simulink model "Robo_Bipede_Contato"  (R2020a)
settings: Solver=ode15s  StartTime=0.0  StopTime=1  MaxStep=1e-4  RelTol=1e-4  AbsTol=1e-5  EnableMultiTasking=on
model workspace: external: MATLAB File C:\Users\LUIS IZQUIERDO C\Desktop\PROGRAMAS TESE\13. ROBO BIPEDE SIMSCAPE COM CONTATO\Model_Params_Contato.m (data not in the file)
values from neighbouring files (symbols this model uses):
  CoG_y = 0.091733    [Model_Params_Cont_FSM.m]
  height_plane = 0.025    [Model_Params_Cont_FSM.m]
  m_esfera = 1    [Model_Params_Cont_FSM.m]
  plane_height = height_plane    (= 0.025)    [Model_Params_Cont_FSM.m]
  plane_length = 50    [Model_Params_Cont_FSM.m]
  plane_width = 3    [Model_Params_Cont_FSM.m]
  temp = Dados_XY1_D(ciclo,1)    [Model_Params_Cont_FSM.m]
  velocidade = 1    [Model_Params_Cont_FSM.m]
  Xpq2_D = Xpq2_D'    [Model_Params_Cont_FSM.m]
  Xpq3_D = Xpq3_D'    [Model_Params_Cont_FSM.m]
  Ypq2_D = Ypq2_D'    [Model_Params_Cont_FSM.m]
  Ypq3_D = Ypq3_D'    [Model_Params_Cont_FSM.m]
undefined symbols (not defined in the file or in its folder): COXA, HAT, PE, PERNA, X, Y, Z
libraries: nesl_utility x70, sm_lib x61, simulink x1
(part 3 of 3)

== stateflow chart Robo_Bipede_Contato/Chart ==
  settings: updateMethod=DISCRETE  sampleTime=0.002
  state FSM4EV/
    entry:
    theta0_right=[deg2rad(25.6131); deg2rad(14.72863); deg2rad(0.0003)];
    theta0_left=[deg2rad(-9.8611); deg2rad(25.8751); deg2rad(12.74498)];
    Count=1;
    HS1E=0;
    TO1D=0;
    HS2D=0;
    TO2E=0;
    during:
    if Count ~= 100
    Count = Count +1
    else
    Count = 1;
    end
    state ADBE/
      during:
      XqpD = Trajectory1(1,Count) - Trajectory1(3,Count);
      YqpD = Trajectory1(2,Count) - Trajectory1(4,Count);
      XpqE = Trajectory1(7,Count) - Trajectory1(5,Count);
      YpqE = Trajectory1(8,Count) - Trajectory1(6,Count);
      Traj_STR = [ XqpD; YqpD;0];
      Traj_SW = [XpqE; YpqE;0];
      theta_right=Inv_Kinem_Stance(Traj_STR, theta0_right);
      theta_left=Inv_Kinem_Swing(Traj_SW, theta0_left);
      theta0_right=theta_right;
      theta0_left=theta_left;
      if Count==45
      HS1E=1;
      TO2E=0;
      end
    state ADE/
      during:
      XqpD = Trajectory1(1,Count) - Trajectory1(3,Count);
      YqpD = Trajectory1(2,Count)  - Trajectory1(4,Count);
      XqpE = Trajectory1(5,Count) - Trajectory1(7,Count);
      YqpE = Trajectory1(6,Count) - Trajectory1(8,Count);
      Traj_STR=[ XqpD; YqpD;0];
      Traj_STL=[XqpE;  YqpE;0];
      theta_right=Inv_Kinem_Stance(Traj_STR,theta0_right);
      theta_left=Inv_Kinem_Stance(Traj_STL,theta0_left);
      theta0_right=theta_right;
      theta0_left=theta_left;
      if Count==54
      TO1D=1;
      HS1E=0;
      end
    state BDAE/
      during:
      XpqD = Trajectory1(3,Count) - Trajectory1(1,Count);
      YpqD = Trajectory1(4,Count) - Trajectory1(2,Count);
      XqpE = Trajectory1(5,Count) - Trajectory1(7,Count);
      YqpE = Trajectory1(6,Count) - Trajectory1(8,Count);
      Traj_SW = [XpqD;  YpqD;0];
      Traj_STL=[ XqpE; YqpE;0];
      theta_right=Inv_Kinem_Swing(Traj_SW,theta0_right);
      theta_left=Inv_Kinem_Stance(Traj_STL,theta0_left);
      theta0_right=theta_right;
      theta0_left=theta_left;
      if Count==97
      HS2D=1;
      TO1D=0;
      end
    state ADD/
      during:
      XqpD = Trajectory1(1,Count) - Trajectory1(3,Count);
      YqpD = Trajectory1(2,Count)  - Trajectory1(4,Count);
      XqpE = Trajectory1(5,Count) - Trajectory1(7,Count);
      YqpE = Trajectory1(6,Count) - Trajectory1(8,Count);
      Traj_STR=[ XqpD; YqpD;0];
      Traj_STL=[XqpE;  YqpE;0];
      theta_right=Inv_Kinem_Stance(Traj_STR,theta0_right);
      theta_left=Inv_Kinem_Stance(Traj_STL,theta0_left);
      theta0_right=theta_right;
      theta0_left=theta_left;
      if Count==100
      TO2E=1;
      HS2D=0;
      end
    (default) -> ADBE
    ADBE -> ADE : [HS1E==1]
    ADD -> ADBE : [TO2E==1]
    ADE -> BDAE : [TO1D==1]
    BDAE -> ADD : [HS2D==1]
  (default) -> FSM4EV
  data: Ptraj function_input; theta_ini function_input; theta_swing function_output; Ptraj function_input; theta_ini function_input; theta_stance function_output; tempo input; Trajectory1 input; Trajectory2 input; Trajectory3 input; Count local; V input; HS1E local double; TO1D local double; HS2D local double; TO2E local double; XqtD local double; YqtD local double; XtqD local double; YtqD local double; XtqE local double; YtqE local double; XqtE local double; YqtE local double; Traj_SW local size=[3,1]; Traj_STR local size=[3,1]; Traj_STL local size=[3,1]; theta_right output size=[3,1]; theta_left output size=[3,1]; theta0_right local size=[3,1]; theta0_left local size=[3,1]; XpqD local; XpqE local; XqpD local; XqpE local; YpqD local; YpqE local; YqpD local; YqpE local; FcDi input; Pospe_Di input; FcEi input; Pospe_Ei input; ChartMode output Enum: ChartModeType
  function theta_swing = Inv_Kinem_Swing(Ptraj,theta_ini):
    | function theta_swing = Inv_Kinem_Swing(Ptraj,theta_ini)
    | 
    | %% CINEMÁTICA INVERSA PARA A FASE DE BALANCO
    | 
    | Lc = 0.42;     % Comprimento coxa (m)
    | Lj = 0.46;     % Comprimento da perna (m)
    | % Lp = 0.153;  % Comprimento do pe(m) 
    | Lp = 0.10;     % Comprimento do pe(m)
    | H = 1.72;      % Altura da pessoa
    | a0 = 0;
    | d0 = 0.19*H/2; % metade da largura do HAT
    | 
    | % Vetor de angulos iniciais theta_ini = [theta_q; theta_j]
    | theta_q = theta_ini(1);
    | theta_j = theta_ini(2);
    | theta_t = theta_ini(3);
    | 
    | %% EQUACOES DA CINEMATICA DIRETA
    | %Posicao do dedao em relacao a junta do quadril (FASE BALANCO)
    | P_ini =[Lc*sin(theta_q) + Lj*sin(theta_q - theta_j) + Lp*cos(theta_q - theta_j + theta_t); 
    |        -Lc*cos(theta_q) - Lj*cos(theta_q - theta_j) + Lp*sin(theta_q - theta_j + theta_t); 
    |         0];
    | 
    | 
    | %% EQUACOES DA CINEMATICA INVERSA
    | %Matriz Jacobiana Inversa J^-1 Fase de Balanco
    | % determ = Lc*Lj*sj;
    | % Jinv = (1/determ)*[-Lj*sqj, Lj*cqj; -(Lc*sq+Lj*sqj), Lc*cq+Lj*cqj];
    | 
    | tht_1 = theta_q;
    | tht_2 = theta_j;
    | tht_3 = theta_t;
    | 
    | Jinv_bal3gl = zeros(3,3);
    | 
    | Jinv_bal3gl(1,1) = (Lc*Lj^2*cos(tht_1) + 2*Lc*Lp^2*cos(tht_1) +...
    |     2*Lc*Lp^2*cos(tht_1 - 2*tht_2 + 2*tht_3) + Lj*Lp^2*cos(tht_1 - tht_2 + 2*tht_3) -...
    |     Lc*Lj^2*cos(tht_1 - 2*tht_2) + Lj*Lp^2*cos(tht_1 - tht_2) -...
    |     Lc*Lj*Lp*sin(tht_1 + tht_3) + Lc*Lj*Lp*sin(tht_1 - tht_3) +...
    |     2*Lc*Lj*Lp*sin(tht_1 - 2*tht_2 + tht_3))/(Lc^2*Lj^2 + 2*Lc^2*Lp^2 + 2*Lj^2*Lp^2 +...
    |     2*Lc^2*Lp^2*cos(2*tht_2 - 2*tht_3) - Lc^2*Lj^2*cos(2*tht_2) + 2*Lj^2*Lp^2*cos(2*tht_3) -...
    |     2*Lc^2*Lj*Lp*sin(2*tht_2 - tht_3) + 2*Lc*Lj*Lp^2*cos(tht_2) - 2*Lc^2*Lj*Lp*sin(tht_3) +...
    |     2*Lc*Lj*Lp^2*cos(tht_2 - 2*tht_3));
    | 
    | Jinv_bal3gl(2,1) = (Lc^2*Lj*cos(tht_1 + tht_2) + Lc*Lj^2*cos(tht_1) + Lc*Lp^2*cos(tht_1) +...
    |     Lc*Lp^2*cos(tht_1 - 2*tht_2 + 2*tht_3) - Lj*Lp^2*cos(tht_1 - tht_2 + 2*tht_3) -...
    |     Lc^2*Lj*cos(tht_1 - tht_2) - Lc*Lj^2*cos(tht_1 - 2*tht_2) - Lj*Lp^2*cos(tht_1 - tht_2) +...
    |     Lc^2*Lp*sin(tht_1 + tht_2 - tht_3) + Lc^2*Lp*sin(tht_1 - tht_2 + tht_3) -...
    |     Lc*Lj*Lp*sin(tht_1 + tht_3) + Lc*Lj*Lp*sin(tht_1 - tht_3) +...
    |     2*Lc*Lj*Lp*sin(tht_1 - 2*tht_2 + tht_3))/(Lc^2*Lj^2 + 2*Lc^2*Lp^2 + 2*Lj^2*Lp^2 +...
    |     2*Lc^2*Lp^2*cos(2*tht_2 - 2*tht_3) - Lc^2*Lj^2*cos(2*tht_2) + 2*Lj^2*Lp^2*cos(2*tht_3) -...
    |     2*Lc^2*Lj*Lp*sin(2*tht_2 - tht_3) + 2*Lc*Lj*Lp^2*cos(tht_2) - 2*Lc^2*Lj*Lp*sin(tht_3) +...
    |     2*Lc*Lj*Lp^2*cos(tht_2 - 2*tht_3));
    | 
    | Jinv_bal3gl(3,1) = -(Lp*(Lc^2*sin(tht_1 + tht_2 - tht_3) + Lc^2*sin(tht_1 - tht_2 + tht_3) +...
    |     2*Lj^2*sin(tht_1 - tht_2 + tht_3) - 2*Lj^2*sin(tht_2 - tht_1 + tht_3) +...
    |     2*Lj*Lp*cos(tht_1 - tht_2) + 2*Lc*Lj*sin(tht_1 - tht_3) +...
    |     Lc*Lj*sin(tht_1 - 2*tht_2 + tht_3) + Lc*Lj*sin(tht_1 + tht_3) +...
    |     Lc*Lp*cos(tht_1) + Lc*Lp*cos(tht_1 - 2*tht_2 + 2*tht_3) +...
    |     2*Lj*Lp*cos(tht_1 - tht_2 + 2*tht_3)))/(Lc^2*Lj^2 + 2*Lc^2*Lp^2 +...
    |     2*Lj^2*Lp^2 + 2*Lc^2*Lp^2*cos(2*tht_2 - 2*tht_3) - Lc^2*Lj^2*cos(2*tht_2) +...
    |     2*Lj^2*Lp^2*cos(2*tht_3) - 2*Lc^2*Lj*Lp*sin(2*tht_2 - tht_3) +...
    |     2*Lc*Lj*Lp^2*cos(tht_2) - 2*Lc^2*Lj*Lp*sin(tht_3) + 2*Lc*Lj*Lp^2*cos(tht_2 - 2*tht_3));
    | 
    | Jinv_bal3gl(1,2) = (Lc*Lj^2*sin(tht_1) + 2*Lc*Lp^2*sin(tht_1) +...
    |     2*Lc*Lp^2*sin(tht_1 - 2*tht_2 + 2*tht_3) + Lj*Lp^2*sin(tht_1 - tht_2 + 2*tht_3) -...
    |     Lc*Lj^2*sin(tht_1 - 2*tht_2) + Lj*Lp^2*sin(tht_1 - tht_2) -...
    |     Lc*Lj*Lp*cos(tht_1 - tht_3) - 2*Lc*Lj*Lp*cos(tht_1 - 2*tht_2 + tht_3) +...
    |     Lc*Lj*Lp*cos(tht_1 + tht_3))/(Lc^2*Lj^2 + 2*Lc^2*Lp^2 + 2*Lj^2*Lp^2 +...
    |     2*Lc^2*Lp^2*cos(2*tht_2 - 2*tht_3) - Lc^2*Lj^2*cos(2*tht_2) + 2*Lj^2*Lp^2*cos(2*tht_3) -...
    |     2*Lc^2*Lj*Lp*sin(2*tht_2 - tht_3) + 2*Lc*Lj*Lp^2*cos(tht_2) - 2*Lc^2*Lj*Lp*sin(tht_3) +...
    |     2*Lc*Lj*Lp^2*cos(tht_2 - 2*tht_3));
    | 
    | Jinv_bal3gl(2,2) = -(Lj*Lp^2*sin(tht_1 - tht_2 + 2*tht_3) - Lc*Lj^2*sin(tht_1) -...
    |     Lc*Lp^2*sin(tht_1) - Lc*Lp^2*sin(tht_1 - 2*tht_2 + 2*tht_3) - Lc^2*Lj*sin(tht_1 +...
    |     tht_2) + Lc^2*Lj*sin(tht_1 - tht_2) + Lc*Lj^2*sin(tht_1 - 2*tht_2) +...
    |     Lj*Lp^2*sin(tht_1 - tht_2) + Lc^2*Lp*cos(tht_1 + tht_2 - tht_3) +...
    |     Lc^2*Lp*cos(tht_1 - tht_2 + tht_3) + Lc*Lj*Lp*cos(tht_1 - tht_3) +...
    |     2*Lc*Lj*Lp*cos(tht_1 - 2*tht_2 + tht_3) -...
    |     Lc*Lj*Lp*cos(tht_1 + tht_3))/(Lc^2*Lj^2 + 2*Lc^2*Lp^2 + 2*Lj^2*Lp^2 +...
    |     2*Lc^2*Lp^2*cos(2*tht_2 - 2*tht_3) - Lc^2*Lj^2*cos(2*tht_2) +...
    |     2*Lj^2*Lp^2*cos(2*tht_3) - 2*Lc^2*Lj*Lp*sin(2*tht_2 - tht_3) +...
    |     2*Lc*Lj*Lp^2*cos(tht_2) - 2*Lc^2*Lj*Lp*sin(tht_3) + 2*Lc*Lj*Lp^2*cos(tht_2 - 2*tht_3));
    | 
    | Jinv_bal3gl(3,2) = (Lp*(Lc^2*cos(tht_1 + tht_2 - tht_3) + Lc^2*cos(tht_1 - tht_2 + tht_3) +...
    |     2*Lj^2*cos(tht_1 - tht_2 + tht_3) + 2*Lj^2*cos(tht_2 - tht_1 + tht_3) +...
    |     2*Lc*Lj*cos(tht_1 - tht_3) - 2*Lj*Lp*sin(tht_1 - tht_2) +...
    |     Lc*Lj*cos(tht_1 - 2*tht_2 + tht_3) + Lc*Lj*cos(tht_1 + tht_3) - Lc*Lp*sin(tht_1) -...
    |     Lc*Lp*sin(tht_1 - 2*tht_2 + 2*tht_3) - 2*Lj*Lp*sin(tht_1 - tht_2 + 2*tht_3)))/(Lc^2*Lj^2 +...
    |     2*Lc^2*Lp^2 + 2*Lj^2*Lp^2 + 2*Lc^2*Lp^2*cos(2*tht_2 - 2*tht_3) - Lc^2*Lj^2*cos(2*tht_2) +...
    |     2*Lj^2*Lp^2*cos(2*tht_3) - 2*Lc^2*Lj*Lp*sin(2*tht_2 - tht_3) + 2*Lc*Lj*Lp^2*cos(tht_2) -...
    |     2*Lc^2*Lj*Lp*sin(tht_3) + 2*Lc*Lj*Lp^2*cos(tht_2 - 2*tht_3));
    | 
    | Jinv_bal3gl(1,3) = 0;
    | Jinv_bal3gl(2,3) = 0;
    | Jinv_bal3gl(3,3) = 0;
    | 
    | % Delta de posicao [Xtraj-X_ini; Ytraj-Y_ini, Ztraj - Z_ini];
    | % Ptraj(3) = 0;
    | Delta_P = Ptraj - P_ini;
    | 
    | % Delta_theta = Jinv*Delta_P;
    | Delta_theta = Jinv_bal3gl*Delta_P;
    | 
    | theta_swing = theta_ini + Delta_theta;
  function theta_stance = Inv_Kinem_Stance(Ptraj,theta_ini):
    | function theta_stance = Inv_Kinem_Stance(Ptraj,theta_ini)
    | 
    | %% CINEMÁTICA INVERSA PARA A FASE DE APOIO
    | Lc = 0.42;    % Comprimento coxa (m)
    | Lj = 0.46;    % Comprimento da perna (m)
    | Lp = 0.11;    % Comprimento do pe(m)
    | H = 1.72;     % Altura da pessoa
    | % a0 = 0.16*H/2; % metade da altura do HAT
    | a0 = 0;
    | d0 = 0.19*H/2; % metade da largura do HAT
    | 
    | % Vetor de angulos iniciais theta_ini = [theta_q; theta_j, theta_t]
    | theta_q = theta_ini(1);
    | theta_j = theta_ini(2);
    | theta_t = theta_ini(3);
    | 
    | tht_q = theta_q;
    | tht_j = theta_j;
    | tht_t = theta_t;
    | %Posicao do quadril em relacao a junta do tornozelo (FASE APOIO)
    | % P_ini = [-Lj*sqj-Lc*sq; Lj*cqj+Lc*cq];
    | %Posicao do quadril em relacao a junta do tornozelo (FASE APOIO)
    | 
    | % Ptraj(3,1) = 0;
    | 
    | P_ini =  [-Lc*sin(tht_q) - Lj*sin(tht_q - tht_j) - Lp*cos(tht_q - tht_j + tht_t);
    |             a0 + Lc*cos(tht_q) + Lj*cos(tht_q - tht_j) - Lp*sin(tht_q - tht_j + tht_t);
    |             0];
    | 
    | % CÁLCULO DA MATRIZ JACOBIANA INVERSA PARA A FASE DE APOIO COM A
    | % REFERENCIA O0X0Y0Z0 NO DEDAO E END-EFFECTOR NO CoM DO HAT
    | Jinv_A3gl = zeros(3,3);
    | 
    | Jinv_A3gl(1,1) = -(Lc*Lj^2*cos(tht_q) + 2*Lc*Lp^2*cos(tht_q) +...
    |     2*Lc*Lp^2*cos(tht_q - 2*tht_j + 2*tht_t) + Lj*Lp^2*cos(tht_q - tht_j + 2*tht_t) +...
    |     Lj*Lp^2*cos(tht_j - tht_q) - Lc*Lj^2*cos(2*tht_j - tht_q) - Lc*Lj*Lp*sin(tht_q + tht_t) +...
    |     Lc*Lj*Lp*sin(tht_q - tht_t) + 2*Lc*Lj*Lp*sin(tht_q - 2*tht_j + tht_t))/(Lc^2*Lj^2 +...
    |     2*Lc^2*Lp^2 + 2*Lj^2*Lp^2 + 2*Lc^2*Lp^2*cos(2*tht_j - 2*tht_t) - Lc^2*Lj^2*cos(2*tht_j) +...
    |     2*Lj^2*Lp^2*cos(2*tht_t) - 2*Lc^2*Lj*Lp*sin(2*tht_j - tht_t) +...
    |     2*Lc*Lj*Lp^2*cos(tht_j) - 2*Lc^2*Lj*Lp*sin(tht_t) + 2*Lc*Lj*Lp^2*cos(tht_j - 2*tht_t));
    | 
    | Jinv_A3gl(1,2) = -(Lc*Lj^2*sin(tht_q) + 2*Lc*Lp^2*sin(tht_q) +...
    |     2*Lc*Lp^2*sin(tht_q - 2*tht_j + 2*tht_t) +...
    |     Lj*Lp^2*sin(tht_q - tht_j + 2*tht_t) - Lj*Lp^2*sin(tht_j - tht_q) +...
    |     Lc*Lj^2*sin(2*tht_j - tht_q) - Lc*Lj*Lp*cos(tht_q - tht_t) -...
    |     2*Lc*Lj*Lp*cos(tht_q - 2*tht_j + tht_t) + Lc*Lj*Lp*cos(tht_q + tht_t))/(Lc^2*Lj^2 +...
    |     2*Lc^2*Lp^2 + 2*Lj^2*Lp^2 + 2*Lc^2*Lp^2*cos(2*tht_j - 2*tht_t) - Lc^2*Lj^2*cos(2*tht_j) +...
    |     2*Lj^2*Lp^2*cos(2*tht_t) - 2*Lc^2*Lj*Lp*sin(2*tht_j - tht_t) +...
    |     2*Lc*Lj*Lp^2*cos(tht_j) - 2*Lc^2*Lj*Lp*sin(tht_t) + 2*Lc*Lj*Lp^2*cos(tht_j - 2*tht_t));
    | 
    | Jinv_A3gl(1,3) = 0;
    | 
    | Jinv_A3gl(2,1) = -(Lc^2*Lj*cos(tht_j + tht_q) + Lc*Lj^2*cos(tht_q) + Lc*Lp^2*cos(tht_q) +...
    |     Lc*Lp^2*cos(tht_q - 2*tht_j + 2*tht_t) - Lj*Lp^2*cos(tht_q - tht_j + 2*tht_t) -...
    |     Lc^2*Lj*cos(tht_j - tht_q) - Lj*Lp^2*cos(tht_j - tht_q) - Lc*Lj^2*cos(2*tht_j - tht_q) +...
    |     Lc^2*Lp*sin(tht_j + tht_q - tht_t) + Lc^2*Lp*sin(tht_q - tht_j + tht_t) -...
    |     Lc*Lj*Lp*sin(tht_q + tht_t) + Lc*Lj*Lp*sin(tht_q - tht_t) +...
    |     2*Lc*Lj*Lp*sin(tht_q - 2*tht_j + tht_t))/(Lc^2*Lj^2 + 2*Lc^2*Lp^2 +...
    |     2*Lj^2*Lp^2 + 2*Lc^2*Lp^2*cos(2*tht_j - 2*tht_t) - Lc^2*Lj^2*cos(2*tht_j) +...
    |     2*Lj^2*Lp^2*cos(2*tht_t) - 2*Lc^2*Lj*Lp*sin(2*tht_j - tht_t) +...
    |     2*Lc*Lj*Lp^2*cos(tht_j) - 2*Lc^2*Lj*Lp*sin(tht_t) + 2*Lc*Lj*Lp^2*cos(tht_j - 2*tht_t));
    | 
    | Jinv_A3gl(2,2) = -(Lc^2*Lj*sin(tht_j + tht_q) + Lc*Lj^2*sin(tht_q) + Lc*Lp^2*sin(tht_q) +...
    |     Lc*Lp^2*sin(tht_q - 2*tht_j + 2*tht_t) - Lj*Lp^2*sin(tht_q - tht_j + 2*tht_t) +...
    |     Lc^2*Lj*sin(tht_j - tht_q) + Lj*Lp^2*sin(tht_j - tht_q) + Lc*Lj^2*sin(2*tht_j - tht_q) -...
    |     Lc^2*Lp*cos(tht_j + tht_q - tht_t) - Lc^2*Lp*cos(tht_q - tht_j + tht_t) -...
    |     Lc*Lj*Lp*cos(tht_q - tht_t) - 2*Lc*Lj*Lp*cos(tht_q - 2*tht_j + tht_t) +...
    |     Lc*Lj*Lp*cos(tht_q + tht_t))/(Lc^2*Lj^2 + 2*Lc^2*Lp^2 + 2*Lj^2*Lp^2 +...
    |     2*Lc^2*Lp^2*cos(2*tht_j - 2*tht_t) - Lc^2*Lj^2*cos(2*tht_j) +...
    |     2*Lj^2*Lp^2*cos(2*tht_t) - 2*Lc^2*Lj*Lp*sin(2*tht_j - tht_t) + 2*Lc*Lj*Lp^2*cos(tht_j) -...
    |     2*Lc^2*Lj*Lp*sin(tht_t) + 2*Lc*Lj*Lp^2*cos(tht_j - 2*tht_t));
    | 
    | Jinv_A3gl(2,3) = 0;
    | % 
    | Jinv_A3gl(3,1) = (Lp*(Lc^2*sin(tht_j + tht_q - tht_t) + Lc^2*sin(tht_q - tht_j + tht_t) -...
    |     2*Lj^2*sin(tht_j - tht_q + tht_t) + 2*Lj^2*sin(tht_q - tht_j + tht_t) +...
    |     2*Lj*Lp*cos(tht_j - tht_q) + 2*Lc*Lj*sin(tht_q - tht_t) + Lc*Lj*sin(tht_q - 2*tht_j + tht_t) +...
    |     Lc*Lj*sin(tht_q + tht_t) + Lc*Lp*cos(tht_q) + Lc*Lp*cos(tht_q - 2*tht_j + 2*tht_t) +...
    |     2*Lj*Lp*cos(tht_q - tht_j + 2*tht_t)))/(Lc^2*Lj^2 + 2*Lc^2*Lp^2 + 2*Lj^2*Lp^2 +...
    |     2*Lc^2*Lp^2*cos(2*tht_j - 2*tht_t) - Lc^2*Lj^2*cos(2*tht_j) + 2*Lj^2*Lp^2*cos(2*tht_t) -...
    |     2*Lc^2*Lj*Lp*sin(2*tht_j - tht_t) + 2*Lc*Lj*Lp^2*cos(tht_j) -...
    |     2*Lc^2*Lj*Lp*sin(tht_t) + 2*Lc*Lj*Lp^2*cos(tht_j - 2*tht_t));
    | 
    | Jinv_A3gl(3,2) = -(Lp*(Lc^2*cos(tht_j + tht_q - tht_t) + Lc^2*cos(tht_q - tht_j + tht_t) +...
    |     2*Lj^2*cos(tht_j - tht_q + tht_t) + 2*Lj^2*cos(tht_q - tht_j + tht_t) +...
    |     2*Lc*Lj*cos(tht_q - tht_t) + 2*Lj*Lp*sin(tht_j - tht_q) + Lc*Lj*cos(tht_q - 2*tht_j + tht_t) +...
    |     Lc*Lj*cos(tht_q + tht_t) - Lc*Lp*sin(tht_q) - Lc*Lp*sin(tht_q - 2*tht_j + 2*tht_t) -...
    |     2*Lj*Lp*sin(tht_q - tht_j + 2*tht_t)))/(Lc^2*Lj^2 + 2*Lc^2*Lp^2 + 2*Lj^2*Lp^2 +...
    |     2*Lc^2*Lp^2*cos(2*tht_j - 2*tht_t) - Lc^2*Lj^2*cos(2*tht_j) +...
    |     2*Lj^2*Lp^2*cos(2*tht_t) - 2*Lc^2*Lj*Lp*sin(2*tht_j - tht_t) +...
    |     2*Lc*Lj*Lp^2*cos(tht_j) - 2*Lc^2*Lj*Lp*sin(tht_t) + 2*Lc*Lj*Lp^2*cos(tht_j - 2*tht_t));
    | 
    | Jinv_A3gl(3,3) = 0;
    | 
    | 
    | % Delta de posicao [Xtraj-X_ini; Ytraj-Y_ini];
    | Delta_P = Ptraj - P_ini;
    | 
    | % Delta theta = J^-1*Delta_p
    | Delta_theta = Jinv_A3gl*Delta_P;
    | 
    | theta_stance = theta_ini + Delta_theta;
